simulink model "boucing_ball"  (R2022b)
settings: Solver=VariableStepAuto  StartTime=0.0  StopTime=20.0  RelTol=1e-3
libraries: vrlib x2
settings Model: Creator=Vivianne  LastModifiedBy=Vivianne

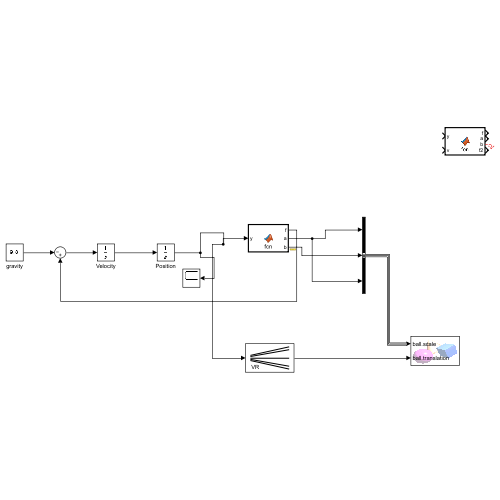
[thumbnail: Simulink's stored preview of the top-level diagram]
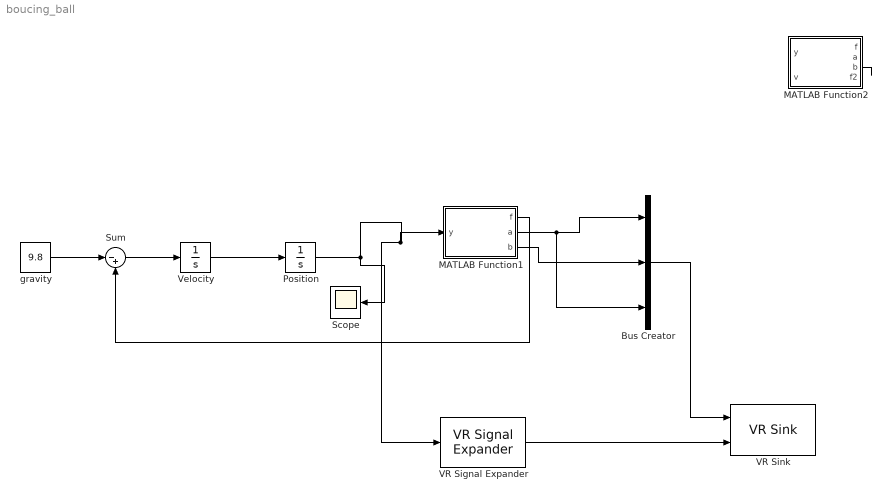
== system boucing_ball ==
  Bus Creator : BusCreator  Inputs=3
  MATLAB Function1 : MATLAB Function  TreatAsAtomicUnit=on
  MATLAB Function2 : MATLAB Function  TreatAsAtomicUnit=on
  Position : Integrator  InitialCondition=20
  Scope : Scope
  Sum : Sum  Inputs=|-+
  VR Signal Expander : vrlib/VR Signal Expander  outwidth=3  outidx=[2]
  VR Sink : vrlib/VR Sink  InstantiateOnLoad=on  SampleTime=0.01  ViewEnable=on  RemoteChange=off  RemoteView=off  FieldsWritten=ball.scale.3.1.1.double#ball.translation.3.1.1.double  WorldFileName=boucing-ball2.x3d  AutoView=off  VideoDimensions=[]  AllowVariableSize=off
  Velocity : Integrator
  gravity : Constant  Value=9.8
  wires:
  Velocity/1 -> Position/1
  Position/1 -> MATLAB Function1/1(y), VR Signal Expander/1, Scope/1
  gravity/1 -> Sum/1
  Sum/1 -> Velocity/1
  MATLAB Function1/1(f) -> Sum/2
  VR Signal Expander/1 -> VR Sink/2
  MATLAB Function1/2(a) -> Bus Creator/3, Bus Creator/1
  Bus Creator/1 -> VR Sink/1
  MATLAB Function1/3(b) -> Bus Creator/2
  MATLAB Function2/3(b) -> ?

== matlab function boucing_ball/MATLAB Function1 ==
  data: y input; f output; a output; b output
function [f, a, b] = fcn(y)
%#eml

if y<1e-4;
    y=1e-4
end

if y<1.5
    f=500*(1.5-y)
    a=sqrt(1.5^3/y);
    b=y;
else 
    f=0;
    a=1.5;
    b=1.5
end

== matlab function boucing_ball/MATLAB Function2 ==
  data: y input; f output; v input; a output; b output; f2 output
function [f, a, b, f2] = fcn(y, v)
%#eml
f2=0;
if y<1e-4
 y=1e-4;
end

if y<1.5
    f1=500*(1.5-y);
    if v<0
        f2=-10*v;
    end
    a=sqrt(1.5^3/y);
    b=y;
else 
    f1=0;
    a=1.5;
    b=1.5;
end
f=f1+f2;
